simulink model "Todo_EKF_1er_Riccati2014"  (R2015a)
settings: Solver=FixedStepDiscrete  StartTime=0.0  StopTime=60  FixedStep=0.02  RelTol=1e-3
InitFcn:
  | load('Pose_integration_R_L.mat')
  | ProcNoiseD=0.01^2; % is a variance
  | ProcNoiseTheta=0.001^2; % is a variance
StopFcn:
  | I = imread('Enviroment.png');
  | x = [0 35.9];
  | y=[23.31 0];
  | image(I,'XData',x,'YData',y);
  | axis xy;
  | hold on
  | plot (Pose_t.Data(:,1),Pose_t.Data(:,2),'b');
  | plot (Pose_est.Data(:,1),Pose_est.Data(:,2),'r');
  | len=length(Pose_t.Data);
  | for i=1:round(len/15):len
  | %    plot_ellipse(Pk.signals.values(1:2,1:2,i),[xEst.signals.values(i,1), xEst.signals.values(i,2)],'g');
  |     plot_ellipse(Pk.signals.values(1:2,1:2,i),[Pose_est.Data(i,1), Pose_est.Data(i,2)],'g');
  |     title('Todo Deliverable with Odometry Noise with constant V_d and V_\theta but different P\_ini Values');
  | end
settings Model: Creator=antonio  LastModifiedBy=saiki
settings DebuggingCC: UnderspecifiedInitializationDetection=Classic  MergeDetectMultiDrivingBlocksExec=none  SolverPrmCheckMsg=warning  StateNameClashWarn=warning

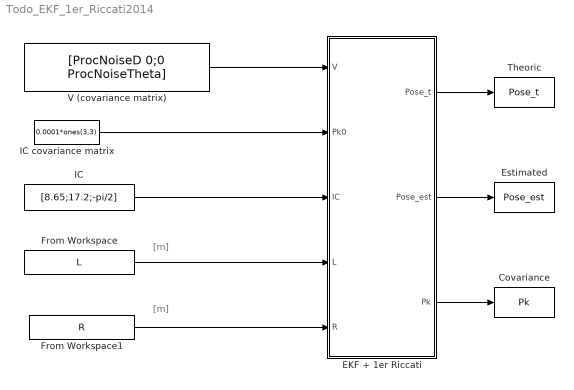
== system Todo_EKF_1er_Riccati2014 ==
  note: [m]
  note: [m]
  Covariance : ToWorkspace  VariableName=Pk  SaveFormat=Structure With Time  SampleTime=-1
  EKF + 1er Riccati : MATLAB Function  TreatAsAtomicUnit=on
  Estimated : ToWorkspace  VariableName=Pose_est  SaveFormat=Timeseries  SampleTime=-1
  From Workspace : FromWorkspace  VariableName=L  SampleTime=0
  From Workspace1 : FromWorkspace  VariableName=R  SampleTime=0
  IC : Constant  Value=[8.65;17.2;-pi/2]
  IC covariance matrix : FromWorkspace  VariableName=0.0001*ones(3,3)
  Theoric : ToWorkspace  VariableName=Pose_t  SaveFormat=Timeseries  SampleTime=-1
  V (covariance matrix) : Constant  Value=[ProcNoiseD 0;0 ProcNoiseTheta]  VectorParams1D=off
  wires:
  IC/1 -> EKF + 1er Riccati/3(IC)
  EKF + 1er Riccati/1(Pose_t) -> Theoric/1
  EKF + 1er Riccati/2(Pose_est) -> Estimated/1
  From Workspace1/1 -> EKF + 1er Riccati/5(R)
  From Workspace/1 -> EKF + 1er Riccati/4(L)
  V (covariance matrix)/1 -> EKF + 1er Riccati/1(V)
  IC covariance matrix/1 -> EKF + 1er Riccati/2(Pk0)
  EKF + 1er Riccati/3(Pk) -> Covariance/1

== matlab function Todo_EKF_1er_Riccati2014/EKF + 1er Riccati ==
  data: V input; Pk0 input; Pose_t output; Pose_est output; IC input; L input; R input; Pk output
function [Pose_t,Pose_est,Pk] = fcn(V,Pk0,IC,L,R) % IC->Initial Condition [xo,yo,th0]
                                   % R and L are the displacements of
                                   % wheels [m]
persistent x_w y_w suma_theta  %  internal variable to be mantain its values
persistent Pose_est1 Pose_t1 Pk1

ts=0.02; % sample time
S = 0.26;

%%%%%%%%%%%%%%%%%%%%%%%%%%%%%%%%%%%%%%%%%%%%%%%%%%%%%%%%%%%%%%%%%%%%%%%%%%
% %%%%%%%%%%%%%%   Read Initial condition   %%%%%%%%%%%%%%%%%%%%%%%%%%%%%%
x_ini=IC(1);
y_ini=IC(2);
theta_ini=IC(3);
P_ini=0.0001*ones(3,3);

% V = diag([0.001^2 0.002^2]);
%%%%%%%%%%%%%%%%%%%%%%%%%%%%%%%%%%%%%%%%%%%%%%%%%%%%%%%%%%%%%%%%%%%%%%%%%%
%%%%%%%%%%%%%%%   variable initialitation  %%%%%%%%%%%%%%%%%%%%%%%%%%%%%%
if isempty (x_w)
    x_w=x_ini;
    y_w=y_ini;
    suma_theta=theta_ini; 
    Pose_est1 = [x_w;y_w;suma_theta];
    Pose_t=[x_w;y_w;suma_theta]
    Pk1 = P_ini;
end
%%%%%%%%%%%%%%%%%%%%%%%%%%%%%%%%%%%%%%%%%%%%%%%%%%%%%%%%%%%%%%%%%%%%%%%%%%
%%%%%%%%%%%%%%%%%  compute the odometry    %%%%%%%%%%%%%%%%%%%%%%%%%%%%%%%
delta_th = ((R-L)/(2*S));
delta_d = (R+L)/2;
%%%%%%%%%%%%%%%%%%%%%%%%%%%%%%%%%%%%%%%%%%%%%%%%%%%%%%%%%%%%%%%%%%%%%%%%%%
%%%%%%%%%%%%%%%%%  integration of the robot pose %%%%%%%%%%%%%%%%%%%%%%%%%%

x_w = x_w + (delta_d + V(1,1))*cos(suma_theta + delta_th + V(2,2))
y_w = y_w + (delta_d + V(1,1))*sin(suma_theta + delta_th + V(2,2))
suma_theta=mod((suma_theta + delta_th + V(2,2)) ,2*pi); 

Pose_t=[x_w;y_w;suma_theta];

%%%%%%%%%%%%%%%%%%%%%%%%%%%%%%%%%%%%%%%%%%%%%%%%%%%%%%%%%%%%%%%%%%%%%%%%%%
%%%%%%%%%%%%%%%%%  Build the Jacocian %%%%%%%%%%%%%%%%%%%%%%%%%%%%%%%%%%%%3

F_x = [[1 0 -(delta_d*sin(suma_theta+delta_th))];....
      [0 1 -(delta_d*cos(suma_theta+delta_th))];....
      [0 0 1]];

F_v = [[cos(suma_theta+delta_th) -delta_d*sin(suma_theta+delta_th)];....
      [sin(suma_theta+delta_th) delta_d*cos(suma_theta+delta_th)];[0 1]];

%%%%%%%%%%%%%%%%%%%%%%%%%%%%%%%%%%%%%%%%%%%%%%%%%%%%%%%%%%%%%%%%%%%%%%%%%%
%%%%%%%%%%%%%%%%% Compute the EKF Trucated Taylor %%%%%%%%%%%%%%%%%%%%%%%%

Pose_est1 = Pose_est1 + F_x*(Pose_t - Pose_est1) + F_v*diag(V);

Pk1 = F_x*Pk1*F_x' + F_v*V*F_v';

%%%%%%%%%%%%%%%%%%%%%%%%%%%%%%%%%%%%%%%%%%%%%%%%%%%%%%%%%%%%%%%%%%%%%%%%%%
%%%%%%%%%%%%%%%%%  output variable %%%%%%%%%%%%%%%%%%%%%%%%%%%%%%%%%%%%%%%

Pose_t=[x_w;y_w;suma_theta]
Pose_est= Pose_est1
Pk=Pk1

end
